simulink model "sum_fft"  (Simulink 7.9)
settings: Solver=ode45  StartTime=0.0  StopTime=Tsim  RelTol=1e-3
values from neighbouring files (symbols this model uses):
  Fsin1 = 85005.9*2*pi    (= 534107.821904)    [somme_fft.m]
  Fsin2 = 90000*2*pi    (= 565486.677646)    [somme_fft.m]
  Fsin3 = 94986.8*2*pi    (= 596819.666136)    [somme_fft.m]
  Fsin4 = 100000*2*pi    (= 628318.530718)    [somme_fft.m]
  Fsin5 = 115015.9*2*pi    (= 722666.212972)    [somme_fft.m]
  Fsin6 = 120000*2*pi    (= 753982.236862)    [somme_fft.m]
  Te = 1/Fe    (= 3.125e-06)    [Bode_partie1.m]    (also in fft_script.m = 0.03125; script.m = 0.03125; script1.m; script2.m)
settings Model: Creator=anakstel  LastModifiedBy=anakstel

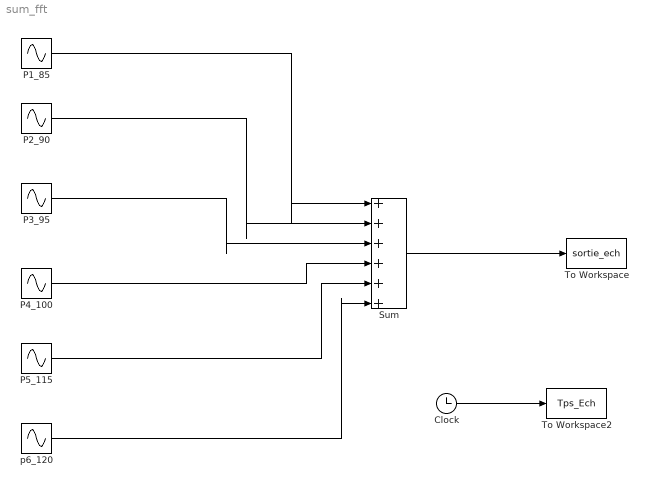
== system sum_fft ==
  Clock : Clock
  P1_85 : Sin  Frequency=Fsin1  SampleTime=0
  P2_90 : Sin  Frequency=Fsin2  SampleTime=0
  P3_95 : Sin  Frequency=Fsin3  SampleTime=0
  P4_100 : Sin  Frequency=Fsin4  SampleTime=0
  P5_115 : Sin  Frequency=Fsin5  SampleTime=0
  Sum : Sum  Inputs=|++++++  SampleTime=Te
  To Workspace : ToWorkspace  VariableName=sortie_ech  SampleTime=Te
  To Workspace2 : ToWorkspace  VariableName=Tps_Ech  SampleTime=Te
  p6_120 : Sin  Frequency=Fsin6  SampleTime=0
  wires:
  P1_85/1 -> Sum/1
  P2_90/1 -> Sum/2
  P3_95/1 -> Sum/3
  P4_100/1 -> Sum/4
  P5_115/1 -> Sum/5
  p6_120/1 -> Sum/6
  Sum/1 -> To Workspace/1
  Clock/1 -> To Workspace2/1
